simulink model "clock_jitter"  (R2025b)
settings: Solver=VariableStepAuto  StartTime=0.0  StopTime=10.0  RelTol=1e-3
settings Model: Creator=divya  LastModifiedBy=divya

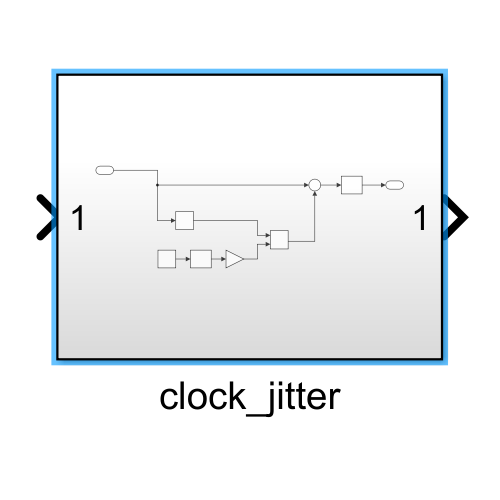
[thumbnail: Simulink's stored preview of the top-level diagram]
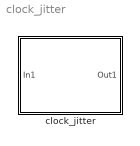
== system clock_jitter ==
  clock_jitter : Subsystem

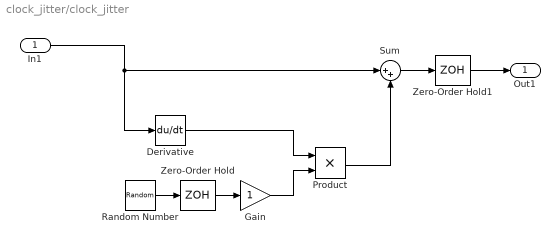
== system clock_jitter/clock_jitter ==
  In1 : Inport
  Derivative : Derivative
  Gain : Gain
  Product : Product
  Random Number : RandomNumber  SampleTime=0.1
  Sum : Sum  Inputs=|++
  Zero-Order Hold : ZeroOrderHold  SampleTime=-1
  Zero-Order Hold1 : ZeroOrderHold  SampleTime=-1
  Out1 : Outport
  wires:
  In1/1 -> Derivative/1, Sum/1
  Derivative/1 -> Product/1
  Zero-Order Hold1/1 -> Out1/1
  Sum/1 -> Zero-Order Hold1/1
  Random Number/1 -> Zero-Order Hold/1
  Product/1 -> Sum/2
  Zero-Order Hold/1 -> Gain/1
  Gain/1 -> Product/2
